simulink subsystem "SimulinkPlantModels"  (R2023a)
settings: Solver=VariableStepAuto  StartTime=0.0  StopTime=10.0  RelTol=1e-3
undefined symbols (not defined in the file): PlntDCDCVoltInit, PlntTrnsfrCaseAxlSpdLock, PlntTrnsfrCaseTrqSplitRatio
libraries: vehdynlibsens x1
(part 2 of 2)

== system SimulinkPlantModels/Sensors/Sensors/IMU Sensor ==
  VehFdbk : Inport
  Bus Creator1 : BusCreator  Inputs=2
  Bus Selector : BusSelector  OutputSignals=BdyFrm.Cg.Acc.ax,BdyFrm.Cg.Acc.ay,BdyFrm.Cg.Acc.az  OutputAsBus=on
  Bus Selector1 : BusSelector  OutputSignals=BdyFrm.Cg.AngVel.p,BdyFrm.Cg.AngVel.q,BdyFrm.Cg.AngVel.r  OutputAsBus=on
  Bus Selector2 : BusSelector  OutputSignals=BdyFrm.Cg.AngAcc.pdot,BdyFrm.Cg.AngAcc.qdot,BdyFrm.Cg.AngAcc.rdot  OutputAsBus=on
  Bus to Vector : BusToVector
  Bus to Vector1 : BusToVector
  Bus to Vector2 : BusToVector
  Constant : Constant  Value=[0,0,0]  SampleTime=-1
  Constant1 : Constant  Value=[0,0,9.81]  SampleTime=-1
  Three-axis Inertial Measurement Unit : vehdynlibsens/Three-axis Inertial Measurement Unit  units=Metric (MKS)  imu=[0 0 0]  i_Ts=0  dtype_a=off  w_a=190  z_a=0.707  a_sf_cc=[1 0 0; 0 1 0; 0 0 1]  a_bias=[0 0 0]  a_sat="[-inf  -inf  -inf  inf inf inf]"  dtype_g=off  w_g=190  z_g=0.707  g_sf_cc=[1 0 0; 0 1 0; 0 0 1]  g_bias=[0 0 0]  g_sens=[0 0 0]  g_sat="[-inf  -inf  -inf  inf inf inf]"  i_rand=on  i_seeds=[23093 23094 23095 23096 23097 23098]  i_pow=[0.001 0.001 0.001 0.0001 0.0001 0.0001]  aMode=2
  Unit Conversion : UnitConversion
  IMU : Outport
  wires:
  VehFdbk/1 -> Bus Selector/1, Bus Selector1/1, Bus Selector2/1
  Constant1/1 -> Three-axis Inertial Measurement Unit/5
  Bus to Vector/1 -> Unit Conversion/1
  Bus Selector1/1 -> Bus to Vector1/1
  Bus to Vector1/1 -> Three-axis Inertial Measurement Unit/2
  Bus Selector/1 -> Bus to Vector/1
  Bus to Vector2/1 -> Three-axis Inertial Measurement Unit/3
  Three-axis Inertial Measurement Unit/1 -> Bus Creator1/1  "Acc"
  Bus Creator1/1 -> IMU/1  "IMU"
  Bus Selector2/1 -> Bus to Vector2/1
  Constant/1 -> Three-axis Inertial Measurement Unit/4
  Three-axis Inertial Measurement Unit/2 -> Bus Creator1/2  "pqr"
  Unit Conversion/1 -> Three-axis Inertial Measurement Unit/1

== system SimulinkPlantModels/Sensors/Sensors/No IMU Sensor ==
  VehFdbk : Inport
  Bus Creator1 : BusCreator  Inputs=2
  Constant : Constant  Value=zeros(3,1)  SampleTime=-1
  Constant1 : Constant  Value=zeros(3,1)  SampleTime=-1
  Terminator : Terminator
  IMU : Outport
  wires:
  VehFdbk/1 -> Terminator/1
  Constant1/1 -> Bus Creator1/2  "pqr"
  Bus Creator1/1 -> IMU/1  "IMU"
  Constant/1 -> Bus Creator1/1  "Acc"

== system SimulinkPlantModels/Drivetrain/Transmission and Actuators/Conventional Vehicle/Transmission ==
  GearCmd : Inport
  EngTrq : Inport  Port=2
  DriveshftSpd : Inport  Port=3
  Automated Manual Transmission : Subsystem  VariantControl=Automated Manual Transmission  ReferencedSubsystem=AutomatedManualTransmission
  Automatic Transmission With Torque Converter : Subsystem  VariantControl=Automatic Transmission With Torque Converter  ReferencedSubsystem=AutomaticTransmissionWithTorqueConverter
  Ideal Fixed Gear Transmission : Subsystem  VariantControl=Ideal Fixed Gear Transmission  ReferencedSubsystem=IdealFixedGearTransmission
  Cltch2State : Outport
  Info : Outport  Port=2
  EngSpd : Outport  Port=3
  DriveshftTrq : Outport  Port=4

== system SimulinkPlantModels/Electrical System/Electrical System/Electric Machines/1EM ==
  EMTrqCmd : Inport
  EMSpd : Inport  Port=2
  BusVolt : Inport  Port=3
  Electric Machine 1 : Subsystem  Variant=on  VariantControlMode=label  LabelModeActiveChoice=Mapped EM
  Motor Coupling Dynamics : TransferFcn  Denominator=[0.01 1]
  Product : Product
  EMTrq : Outport
  EMPwrElec : Outport  Port=2
  EMCurr : Outport  Port=3
  wires:
  Motor Coupling Dynamics/1 -> EMTrq/1  "EMTrq"
  EMTrqCmd/1 -> Electric Machine 1/1(EMTrqCmd)
  BusVolt/1 -> Electric Machine 1/3(BusVolt), Product/2
  Product/1 -> EMPwrElec/1  "EMPwrElec"
  EMSpd/1 -> Electric Machine 1/2(EMSpd)
  Electric Machine 1/2(EMCurr) -> Product/1, EMCurr/1  "EMCurr"
  Electric Machine 1/1(EMTrq) -> Motor Coupling Dynamics/1

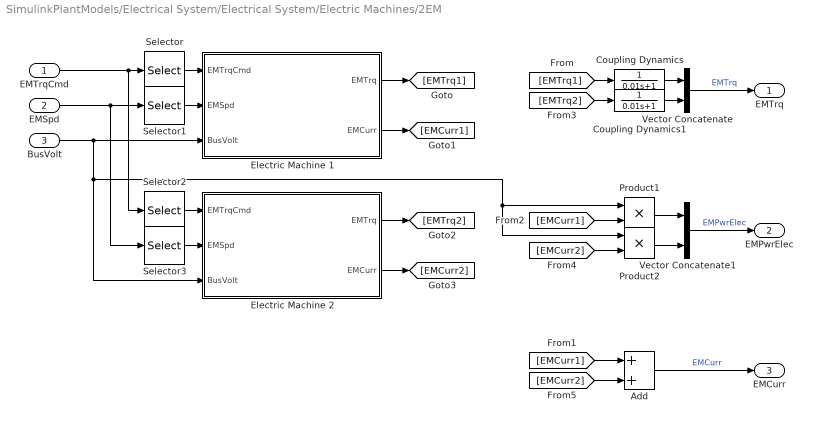
== system SimulinkPlantModels/Electrical System/Electrical System/Electric Machines/2EM ==
  EMTrqCmd : Inport
  EMSpd : Inport  Port=2
  BusVolt : Inport  Port=3
  Add : Sum
  Coupling Dynamics : TransferFcn  Denominator=[0.01 1]
  Coupling Dynamics1 : TransferFcn  Denominator=[0.01 1]
  Electric Machine 1 : Subsystem  Variant=on  VariantControlMode=label  LabelModeActiveChoice=Mapped EM
  Electric Machine 2 : Subsystem  Variant=on  VariantControlMode=label  LabelModeActiveChoice=Mapped EM
  Product1 : Product
  Product2 : Product
  Selector : Selector  InputPortWidth=2  IndexOptions=Index vector (dialog)  Indices=[1]  OutputSizes=1
  Selector1 : Selector  InputPortWidth=2  IndexOptions=Index vector (dialog)  Indices=[1]  OutputSizes=1
  Selector2 : Selector  InputPortWidth=2  IndexOptions=Index vector (dialog)  Indices=[2]  OutputSizes=1
  Selector3 : Selector  InputPortWidth=2  IndexOptions=Index vector (dialog)  Indices=[2]  OutputSizes=1
  Vector Concatenate : Concatenate
  Vector Concatenate1 : Concatenate
  EMTrq : Outport
  EMPwrElec : Outport  Port=2
  EMCurr : Outport  Port=3
  wires:
  Electric Machine 2/2(EMCurr) -> [EMCurr2]
  Electric Machine 2/1(EMTrq) -> [EMTrq2]
  [EMCurr2] -> Add/2
  [EMCurr2] -> Product2/2
  [EMTrq2] -> Coupling Dynamics1/1
  [EMCurr1] -> Product1/2
  [EMCurr1] -> Add/1
  Electric Machine 1/2(EMCurr) -> [EMCurr1]
  [EMTrq1] -> Coupling Dynamics/1
  Electric Machine 1/1(EMTrq) -> [EMTrq1]
  EMSpd/1 -> Selector3/1, Selector1/1
  Selector/1 -> Electric Machine 1/1(EMTrqCmd)
  Add/1 -> EMCurr/1  "EMCurr"
  Selector2/1 -> Electric Machine 2/1(EMTrqCmd)
  Coupling Dynamics1/1 -> Vector Concatenate/2
  Product2/1 -> Vector Concatenate1/2
  Product1/1 -> Vector Concatenate1/1
  EMTrqCmd/1 -> Selector2/1, Selector/1
  Selector3/1 -> Electric Machine 2/2(EMSpd)
  Selector1/1 -> Electric Machine 1/2(EMSpd)
  Vector Concatenate1/1 -> EMPwrElec/1  "EMPwrElec"
  Coupling Dynamics/1 -> Vector Concatenate/1
  BusVolt/1 -> Electric Machine 1/3(BusVolt), Electric Machine 2/3(BusVolt), Product1/1, Product2/1
  Vector Concatenate/1 -> EMTrq/1  "EMTrq"

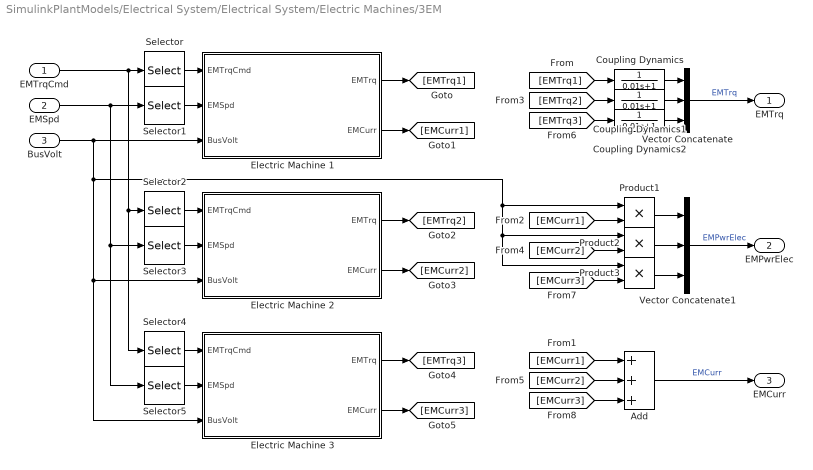
== system SimulinkPlantModels/Electrical System/Electrical System/Electric Machines/3EM ==
  EMTrqCmd : Inport
  EMSpd : Inport  Port=2
  BusVolt : Inport  Port=3
  Add : Sum  Inputs=+++
  Coupling Dynamics : TransferFcn  Denominator=[0.01 1]
  Coupling Dynamics1 : TransferFcn  Denominator=[0.01 1]
  Coupling Dynamics2 : TransferFcn  Denominator=[0.01 1]
  Electric Machine 1 : Subsystem  Variant=on  VariantControlMode=label  LabelModeActiveChoice=Mapped EM
  Electric Machine 2 : Subsystem  Variant=on  VariantControlMode=label  LabelModeActiveChoice=Mapped EM
  Electric Machine 3 : Subsystem  Variant=on  VariantControlMode=label  LabelModeActiveChoice=Mapped EM
  Product1 : Product
  Product2 : Product
  Product3 : Product
  Selector : Selector  InputPortWidth=3  IndexOptions=Index vector (dialog)  Indices=[1]  OutputSizes=1
  Selector1 : Selector  InputPortWidth=3  IndexOptions=Index vector (dialog)  Indices=[1]  OutputSizes=1
  Selector2 : Selector  InputPortWidth=3  IndexOptions=Index vector (dialog)  Indices=[2]  OutputSizes=1
  Selector3 : Selector  InputPortWidth=3  IndexOptions=Index vector (dialog)  Indices=[2]  OutputSizes=1
  Selector4 : Selector  InputPortWidth=3  IndexOptions=Index vector (dialog)  Indices=[3]  OutputSizes=1
  Selector5 : Selector  InputPortWidth=3  IndexOptions=Index vector (dialog)  Indices=[3]  OutputSizes=1
  Vector Concatenate : Concatenate  NumInputs=3
  Vector Concatenate1 : Concatenate  NumInputs=3
  EMTrq : Outport
  EMPwrElec : Outport  Port=2
  EMCurr : Outport  Port=3
  wires:
  [EMTrq3] -> Coupling Dynamics2/1
  Coupling Dynamics2/1 -> Vector Concatenate/3
  Product3/1 -> Vector Concatenate1/3
  [EMCurr3] -> Product3/2
  [EMCurr3] -> Add/3
  Electric Machine 3/2(EMCurr) -> [EMCurr3]
  Electric Machine 3/1(EMTrq) -> [EMTrq3]
  Selector5/1 -> Electric Machine 3/2(EMSpd)
  Selector4/1 -> Electric Machine 3/1(EMTrqCmd)
  Vector Concatenate/1 -> EMTrq/1  "EMTrq"
  BusVolt/1 -> Product2/1, Product3/1, Product1/1, Electric Machine 2/3(BusVolt), Electric Machine 3/3(BusVolt), Electric Machine 1/3(BusVolt)
  Coupling Dynamics/1 -> Vector Concatenate/1
  Vector Concatenate1/1 -> EMPwrElec/1  "EMPwrElec"
  Selector1/1 -> Electric Machine 1/2(EMSpd)
  Selector3/1 -> Electric Machine 2/2(EMSpd)
  EMTrqCmd/1 -> Selector/1, Selector2/1, Selector4/1
  Product1/1 -> Vector Concatenate1/1
  Product2/1 -> Vector Concatenate1/2
  Coupling Dynamics1/1 -> Vector Concatenate/2
  Selector2/1 -> Electric Machine 2/1(EMTrqCmd)
  Add/1 -> EMCurr/1  "EMCurr"
  Selector/1 -> Electric Machine 1/1(EMTrqCmd)
  EMSpd/1 -> Selector1/1, Selector3/1, Selector5/1
  Electric Machine 1/1(EMTrq) -> [EMTrq1]
  [EMTrq1] -> Coupling Dynamics/1
  Electric Machine 1/2(EMCurr) -> [EMCurr1]
  [EMCurr1] -> Add/1
  [EMCurr1] -> Product1/2
  [EMTrq2] -> Coupling Dynamics1/1
  [EMCurr2] -> Product2/2
  [EMCurr2] -> Add/2
  Electric Machine 2/1(EMTrq) -> [EMTrq2]
  Electric Machine 2/2(EMCurr) -> [EMCurr2]

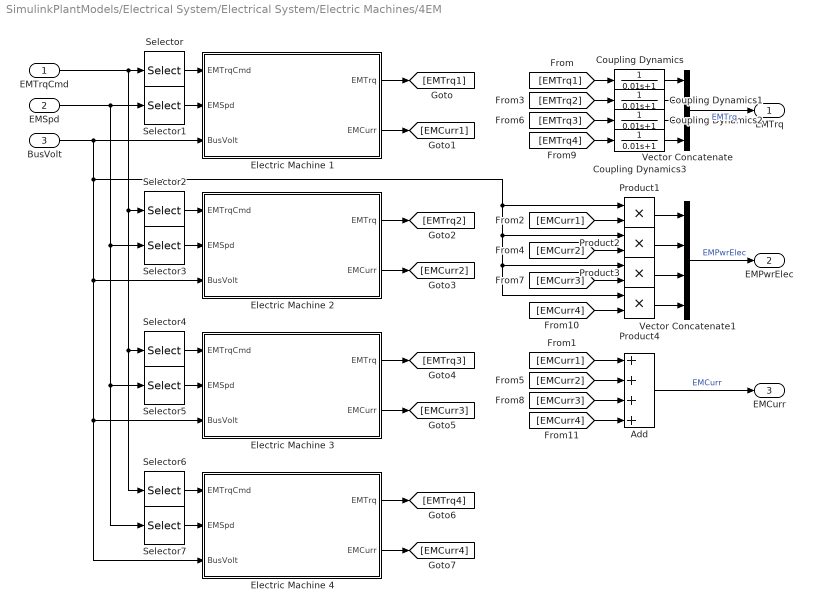
== system SimulinkPlantModels/Electrical System/Electrical System/Electric Machines/4EM ==
  EMTrqCmd : Inport
  EMSpd : Inport  Port=2
  BusVolt : Inport  Port=3
  Add : Sum  Inputs=++++
  Coupling Dynamics{,1..3} (4 alike) : TransferFcn  Denominator=[0.01 1]
  Electric Machine 1 : Subsystem  Variant=on  VariantControlMode=label  LabelModeActiveChoice=Mapped EM
  Electric Machine 2 : Subsystem  Variant=on  VariantControlMode=label  LabelModeActiveChoice=Mapped EM
  Electric Machine 3 : Subsystem  Variant=on  VariantControlMode=label  LabelModeActiveChoice=Mapped EM
  Electric Machine 4 : Subsystem  Variant=on  VariantControlMode=label  LabelModeActiveChoice=Mapped EM
  Product{1..4} (4 alike) : Product
  Selector : Selector  InputPortWidth=4  IndexOptions=Index vector (dialog)  Indices=[1]  OutputSizes=1
  Selector1 : Selector  InputPortWidth=4  IndexOptions=Index vector (dialog)  Indices=[1]  OutputSizes=1
  Selector2 : Selector  InputPortWidth=4  IndexOptions=Index vector (dialog)  Indices=[2]  OutputSizes=1
  Selector3 : Selector  InputPortWidth=4  IndexOptions=Index vector (dialog)  Indices=[2]  OutputSizes=1
  Selector4 : Selector  InputPortWidth=4  IndexOptions=Index vector (dialog)  Indices=[3]  OutputSizes=1
  Selector5 : Selector  InputPortWidth=4  IndexOptions=Index vector (dialog)  Indices=[3]  OutputSizes=1
  Selector6 : Selector  InputPortWidth=4  IndexOptions=Index vector (dialog)  Indices=[4]  OutputSizes=1
  Selector7 : Selector  InputPortWidth=4  IndexOptions=Index vector (dialog)  Indices=[4]  OutputSizes=1
  Vector Concatenate : Concatenate  NumInputs=4
  Vector Concatenate1 : Concatenate  NumInputs=4
  EMTrq : Outport
  EMPwrElec : Outport  Port=2
  EMCurr : Outport  Port=3
  wires:
  [EMCurr4] -> Add/4
  Product4/1 -> Vector Concatenate1/4
  [EMCurr4] -> Product4/2
  [EMTrq4] -> Coupling Dynamics3/1
  Coupling Dynamics3/1 -> Vector Concatenate/4
  Electric Machine 4/2(EMCurr) -> [EMCurr4]
  Electric Machine 4/1(EMTrq) -> [EMTrq4]
  Selector7/1 -> Electric Machine 4/2(EMSpd)
  Selector6/1 -> Electric Machine 4/1(EMTrqCmd)
  Electric Machine 2/2(EMCurr) -> [EMCurr2]
  Electric Machine 2/1(EMTrq) -> [EMTrq2]
  [EMCurr2] -> Add/2
  [EMCurr2] -> Product2/2
  [EMTrq2] -> Coupling Dynamics1/1
  [EMCurr1] -> Product1/2
  [EMCurr1] -> Add/1
  Electric Machine 1/2(EMCurr) -> [EMCurr1]
  [EMTrq1] -> Coupling Dynamics/1
  Electric Machine 1/1(EMTrq) -> [EMTrq1]
  EMSpd/1 -> Selector5/1, Selector7/1, Selector3/1, Selector1/1
  Selector/1 -> Electric Machine 1/1(EMTrqCmd)
  Add/1 -> EMCurr/1  "EMCurr"
  Selector2/1 -> Electric Machine 2/1(EMTrqCmd)
  Coupling Dynamics1/1 -> Vector Concatenate/2
  Product2/1 -> Vector Concatenate1/2
  Product1/1 -> Vector Concatenate1/1
  EMTrqCmd/1 -> Selector6/1, Selector4/1, Selector2/1, Selector/1
  Selector3/1 -> Electric Machine 2/2(EMSpd)
  Selector1/1 -> Electric Machine 1/2(EMSpd)
  Vector Concatenate1/1 -> EMPwrElec/1  "EMPwrElec"
  Coupling Dynamics/1 -> Vector Concatenate/1
  BusVolt/1 -> Electric Machine 1/3(BusVolt), Electric Machine 3/3(BusVolt), Electric Machine 4/3(BusVolt), Electric Machine 2/3(BusVolt), Product1/1, Product4/1, Product3/1, Product2/1
  Vector Concatenate/1 -> EMTrq/1  "EMTrq"
  Selector4/1 -> Electric Machine 3/1(EMTrqCmd)
  Selector5/1 -> Electric Machine 3/2(EMSpd)
  Electric Machine 3/1(EMTrq) -> [EMTrq3]
  Electric Machine 3/2(EMCurr) -> [EMCurr3]
  [EMCurr3] -> Add/3
  [EMCurr3] -> Product3/2
  Product3/1 -> Vector Concatenate1/3
  [EMTrq3] -> Coupling Dynamics2/1
  Coupling Dynamics2/1 -> Vector Concatenate/3

== system SimulinkPlantModels/Electrical System/Electrical System/Electric Machines/1EM/Electric Machine 1 ==
  EMTrqCmd : Inport
  EMSpd : Inport  Port=2
  BusVolt : Inport  Port=3
  Mapped EM : Subsystem  VariantControl=Mapped EM  ReferencedSubsystem=ElectricMachine1
  EMTrq : Outport  VectorParamsAs1DForOutWhenUnconnected=off
  EMCurr : Outport  Port=2  VectorParamsAs1DForOutWhenUnconnected=off

== system SimulinkPlantModels/Electrical System/Electrical System/Electric Machines/2EM/Electric Machine 1 ==
  EMTrqCmd : Inport
  EMSpd : Inport  Port=2
  BusVolt : Inport  Port=3
  Mapped EM : Subsystem  VariantControl=Mapped EM  ReferencedSubsystem=ElectricMachine1
  EMTrq : Outport  VectorParamsAs1DForOutWhenUnconnected=off
  EMCurr : Outport  Port=2  VectorParamsAs1DForOutWhenUnconnected=off

== system SimulinkPlantModels/Electrical System/Electrical System/Electric Machines/2EM/Electric Machine 2 ==
  EMTrqCmd : Inport
  EMSpd : Inport  Port=2
  BusVolt : Inport  Port=3
  Mapped EM : Subsystem  VariantControl=Mapped EM  ReferencedSubsystem=ElectricMachine2
  EMTrq : Outport  VectorParamsAs1DForOutWhenUnconnected=off
  EMCurr : Outport  Port=2  VectorParamsAs1DForOutWhenUnconnected=off

== system SimulinkPlantModels/Electrical System/Electrical System/Electric Machines/3EM/Electric Machine 1 ==
  EMTrqCmd : Inport
  EMSpd : Inport  Port=2
  BusVolt : Inport  Port=3
  Mapped EM : Subsystem  VariantControl=Mapped EM  ReferencedSubsystem=ElectricMachine1
  EMTrq : Outport  VectorParamsAs1DForOutWhenUnconnected=off
  EMCurr : Outport  Port=2  VectorParamsAs1DForOutWhenUnconnected=off

== system SimulinkPlantModels/Electrical System/Electrical System/Electric Machines/3EM/Electric Machine 2 ==
  EMTrqCmd : Inport
  EMSpd : Inport  Port=2
  BusVolt : Inport  Port=3
  Mapped EM : Subsystem  VariantControl=Mapped EM  ReferencedSubsystem=ElectricMachine2
  EMTrq : Outport  VectorParamsAs1DForOutWhenUnconnected=off
  EMCurr : Outport  Port=2  VectorParamsAs1DForOutWhenUnconnected=off

== system SimulinkPlantModels/Electrical System/Electrical System/Electric Machines/3EM/Electric Machine 3 ==
  EMTrqCmd : Inport
  EMSpd : Inport  Port=2
  BusVolt : Inport  Port=3
  Mapped EM : Subsystem  VariantControl=Mapped EM  ReferencedSubsystem=ElectricMachine3
  EMTrq : Outport  VectorParamsAs1DForOutWhenUnconnected=off
  EMCurr : Outport  Port=2  VectorParamsAs1DForOutWhenUnconnected=off

== system SimulinkPlantModels/Electrical System/Electrical System/Electric Machines/4EM/Electric Machine 1 ==
  EMTrqCmd : Inport
  EMSpd : Inport  Port=2
  BusVolt : Inport  Port=3
  Mapped EM : Subsystem  VariantControl=Mapped EM  ReferencedSubsystem=ElectricMachine1
  EMTrq : Outport  VectorParamsAs1DForOutWhenUnconnected=off
  EMCurr : Outport  Port=2  VectorParamsAs1DForOutWhenUnconnected=off

== system SimulinkPlantModels/Electrical System/Electrical System/Electric Machines/4EM/Electric Machine 2 ==
  EMTrqCmd : Inport
  EMSpd : Inport  Port=2
  BusVolt : Inport  Port=3
  Mapped EM : Subsystem  VariantControl=Mapped EM  ReferencedSubsystem=ElectricMachine2
  EMTrq : Outport  VectorParamsAs1DForOutWhenUnconnected=off
  EMCurr : Outport  Port=2  VectorParamsAs1DForOutWhenUnconnected=off

== system SimulinkPlantModels/Electrical System/Electrical System/Electric Machines/4EM/Electric Machine 3 ==
  EMTrqCmd : Inport
  EMSpd : Inport  Port=2
  BusVolt : Inport  Port=3
  Mapped EM : Subsystem  VariantControl=Mapped EM  ReferencedSubsystem=ElectricMachine3
  EMTrq : Outport  VectorParamsAs1DForOutWhenUnconnected=off
  EMCurr : Outport  Port=2  VectorParamsAs1DForOutWhenUnconnected=off

== system SimulinkPlantModels/Electrical System/Electrical System/Electric Machines/4EM/Electric Machine 4 ==
  EMTrqCmd : Inport
  EMSpd : Inport  Port=2
  BusVolt : Inport  Port=3
  Mapped EM : Subsystem  VariantControl=Mapped EM  ReferencedSubsystem=ElectricMachine4
  EMTrq : Outport  VectorParamsAs1DForOutWhenUnconnected=off
  EMCurr : Outport  Port=2  VectorParamsAs1DForOutWhenUnconnected=off
